simulink model "RTdinamic"  (R2018a)
settings: Solver=VariableStepAuto  StartTime=0.0  StopTime=10.0  RelTol=1e-3
settings Model: Creator=ilier  LastModifiedBy=ilier

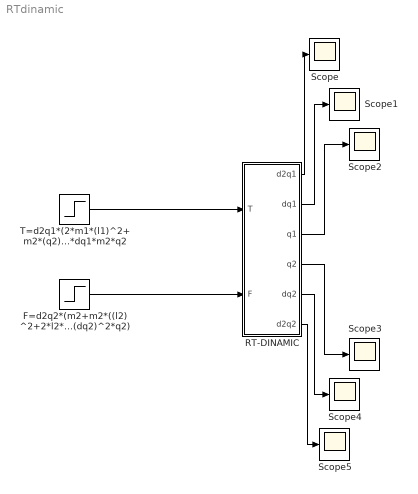
== system RTdinamic ==
  "F=d2q2*(m2+m2*((l2)^2+2*l2*q2+(q2)^2)) -m2*((dq1)^2*q2+(dq2)^2*l2+(dq2)^2*q2) " : Step  SampleTime=0
  RT-DINAMIC : Subsystem
  Scope{,1..5} (6 alike) : Scope
  T=d2q1*(2*m1*(l1)^2+m2*(q2)^2)+2*dq1*m2*q2 : Step  SampleTime=0
  wires:
  T=d2q1*(2*m1*(l1)^2+m2*(q2)^2)+2*dq1*m2*q2/1 -> RT-DINAMIC/1(T)
  "F=d2q2*(m2+m2*((l2)^2+2*l2*q2+(q2)^2)) -m2*((dq1)^2*q2+(dq2)^2*l2+(dq2)^2*q2) "/1 -> RT-DINAMIC/2(F)
  RT-DINAMIC/1(d2q1) -> Scope/1
  RT-DINAMIC/2(dq1) -> Scope1/1
  RT-DINAMIC/3(q1) -> Scope2/1
  RT-DINAMIC/4(q2) -> Scope3/1
  RT-DINAMIC/5(dq2) -> Scope4/1
  RT-DINAMIC/6(d2q2) -> Scope5/1

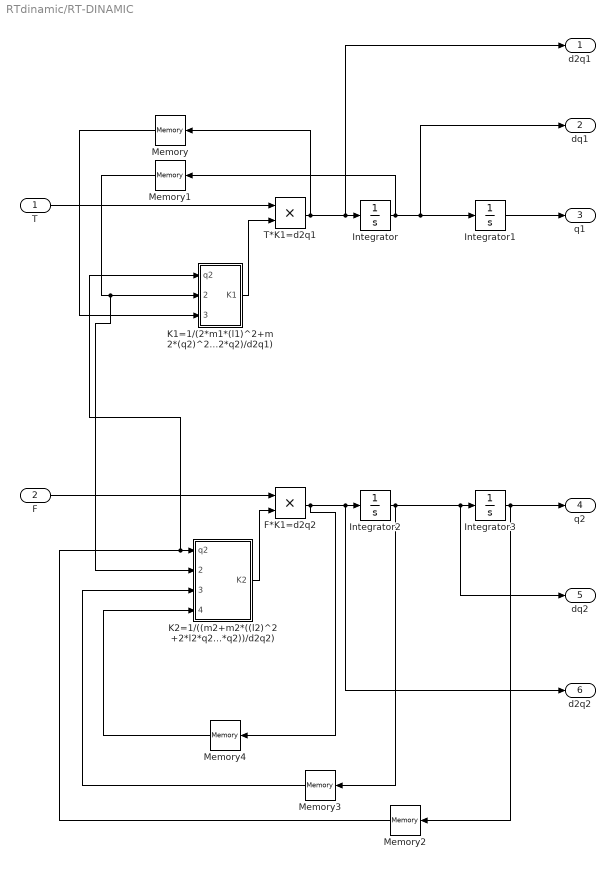
== system RTdinamic/RT-DINAMIC ==
  T : Inport
  F : Inport  Port=2
  F*K1=d2q2 : Product
  Integrator{,1..3} (4 alike) : Integrator
  K1=1/(2*m1*(l1)^2+m2*(q2)^2+(2*dq1*m2*q2)/d2q1) : Subsystem
  K2=1/((m2+m2*((l2)^2+2*l2*q2+(q2)^2)) -(m2*((dq1)^2*q2+(dq2)^2*l2+(dq2)^2*q2))/d2q2) : Subsystem
  Memory{,1..4} (5 alike) : Memory
  T*K1=d2q1 : Product
  d2q1 : Outport
  dq1 : Outport  Port=2
  q1 : Outport  Port=3
  q2 : Outport  Port=4
  dq2 : Outport  Port=5
  d2q2 : Outport  Port=6
  wires:
  F/1 -> F*K1=d2q2/1
  K1=1/(2*m1*(l1)^2+m2*(q2)^2+(2*dq1*m2*q2)/d2q1)/1(K1) -> T*K1=d2q1/2
  T/1 -> T*K1=d2q1/1
  T*K1=d2q1/1 -> Memory/1, d2q1/1, Integrator/1
  Integrator/1 -> Memory1/1, dq1/1, Integrator1/1
  Integrator1/1 -> q1/1
  Memory/1 -> K1=1/(2*m1*(l1)^2+m2*(q2)^2+(2*dq1*m2*q2)/d2q1)/3(d2q1)
  Memory1/1 -> K2=1/((m2+m2*((l2)^2+2*l2*q2+(q2)^2)) -(m2*((dq1)^2*q2+(dq2)^2*l2+(dq2)^2*q2))/d2q2)/2(derivQ1), K1=1/(2*m1*(l1)^2+m2*(q2)^2+(2*dq1*m2*q2)/d2q1)/2(dq1)
  K2=1/((m2+m2*((l2)^2+2*l2*q2+(q2)^2)) -(m2*((dq1)^2*q2+(dq2)^2*l2+(dq2)^2*q2))/d2q2)/1(K2) -> F*K1=d2q2/2
  F*K1=d2q2/1 -> Memory4/1, d2q2/1, Integrator2/1
  Integrator2/1 -> Memory3/1, dq2/1, Integrator3/1
  Integrator3/1 -> Memory2/1, q2/1
  Memory2/1 -> K1=1/(2*m1*(l1)^2+m2*(q2)^2+(2*dq1*m2*q2)/d2q1)/1("q2 "), K2=1/((m2+m2*((l2)^2+2*l2*q2+(q2)^2)) -(m2*((dq1)^2*q2+(dq2)^2*l2+(dq2)^2*q2))/d2q2)/1(q2)
  Memory3/1 -> K2=1/((m2+m2*((l2)^2+2*l2*q2+(q2)^2)) -(m2*((dq1)^2*q2+(dq2)^2*l2+(dq2)^2*q2))/d2q2)/3(derivQ2)
  Memory4/1 -> K2=1/((m2+m2*((l2)^2+2*l2*q2+(q2)^2)) -(m2*((dq1)^2*q2+(dq2)^2*l2+(dq2)^2*q2))/d2q2)/4(deriv2Q2)

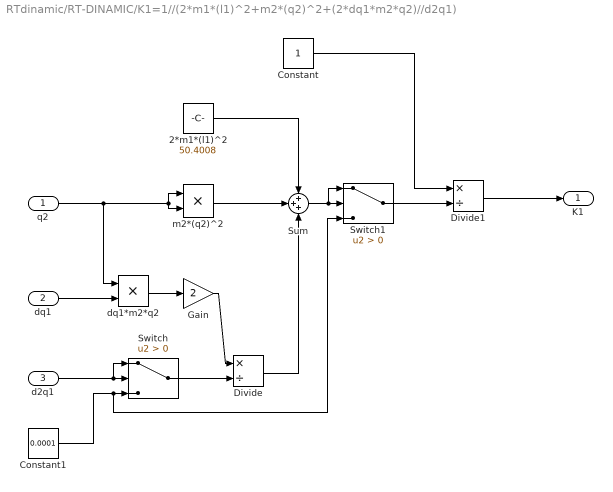
== system RTdinamic/RT-DINAMIC/K1=1//(2*m1*(l1)^2+m2*(q2)^2+(2*dq1*m2*q2)//d2q1) ==
  "q2 " : Inport
  dq1 : Inport  Port=2
  d2q1 : Inport  Port=3
  2*m1*(l1)^2 : Constant  Value=50.4008
  Constant : Constant
  Constant1 : Constant  Value=0.0001
  Divide : Product  Inputs=*/
  Divide1 : Product  Inputs=*/
  Gain : Gain  Gain=2
  Sum : Sum  Inputs=+++
  Switch : Switch  Criteria=u2 > Threshold
  Switch1 : Switch  Criteria=u2 > Threshold
  dq1*m2*q2 : Product
  m2*(q2)^2 : Product
  K1 : Outport
  wires:
  "q2 "/1 -> dq1*m2*q2/1, m2*(q2)^2/2, m2*(q2)^2/1
  2*m1*(l1)^2/1 -> Sum/1
  Sum/1 -> Switch1/1, Switch1/2
  m2*(q2)^2/1 -> Sum/2
  Divide/1 -> Sum/3
  dq1/1 -> dq1*m2*q2/2
  dq1*m2*q2/1 -> Gain/1
  Constant/1 -> Divide1/1
  Gain/1 -> Divide/1
  Divide1/1 -> K1/1
  Switch/1 -> Divide/2
  d2q1/1 -> Switch/1, Switch/2
  Constant1/1 -> Switch1/3, Switch/3
  Switch1/1 -> Divide1/2

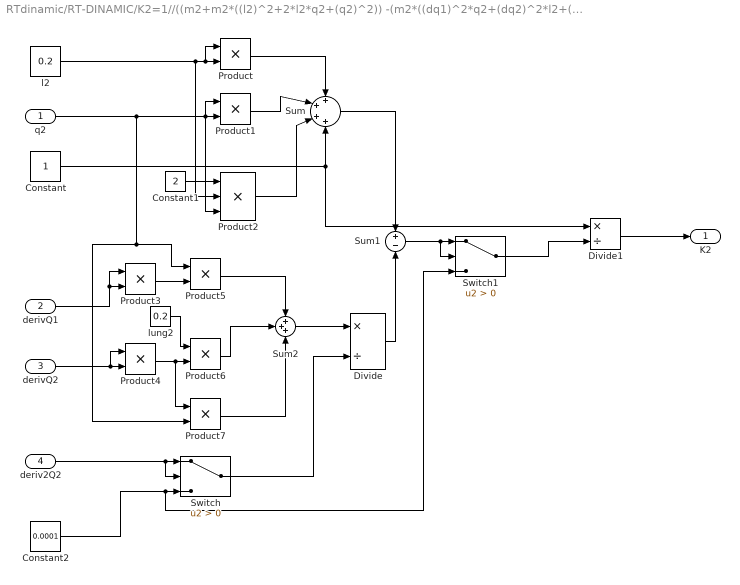
== system RTdinamic/RT-DINAMIC/K2=1//((m2+m2*((l2)^2+2*l2*q2+(q2)^2)) -(m2*((dq1)^2*q2+(dq2)^2*l2+(dq2)^2*q2))//d2q2) ==
  q2 : Inport
  derivQ1 : Inport  Port=2
  derivQ2 : Inport  Port=3
  deriv2Q2 : Inport  Port=4
  Constant : Constant
  Constant1 : Constant  Value=2
  Constant2 : Constant  Value=0.0001
  Divide : Product  Inputs=*/
  Divide1 : Product  Inputs=*/
  Product{,1,3..7} (7 alike) : Product
  Product2 : Product  Inputs=3
  Sum : Sum  Inputs=++++
  Sum1 : Sum  Inputs=+-
  Sum2 : Sum  Inputs=+++
  Switch : Switch  Criteria=u2 > Threshold
  Switch1 : Switch  Criteria=u2 > Threshold
  l2 : Constant  Value=0.2
  lung2 : Constant  Value=0.2
  K2 : Outport
  wires:
  Product5/1 -> Sum2/1
  q2/1 -> Product5/1, Product7/2, Product1/1, Product1/2, Product2/3
  Product1/1 -> Sum/2
  Sum2/1 -> Divide/1
  derivQ1/1 -> Product3/2, Product3/1
  Product4/1 -> Product7/1, Product6/2
  Product6/1 -> Sum2/2
  deriv2Q2/1 -> Switch/2, Switch/1
  l2/1 -> Product/1, Product/2, Product2/2
  Product7/1 -> Sum2/3
  Sum/1 -> Sum1/1
  Divide/1 -> Sum1/2
  Divide1/1 -> K2/1
  derivQ2/1 -> Product4/1, Product4/2
  Constant/1 -> Divide1/1, Sum/4
  lung2/1 -> Product6/1
  Constant1/1 -> Product2/1
  Product3/1 -> Product5/2
  Switch/1 -> Divide/2
  Product/1 -> Sum/1
  Constant2/1 -> Switch1/3, Switch/3
  Product2/1 -> Sum/3
  Sum1/1 -> Switch1/2, Switch1/1
  Switch1/1 -> Divide1/2
